simulink model "main"  (R2022b)
settings: Solver=FixedStepDiscrete  StartTime=0.0  StopTime=2000  FixedStep=0.1  RelTol=1e-3
libraries: simulink x3
settings Model: Creator=86134  LastModifiedBy=86134

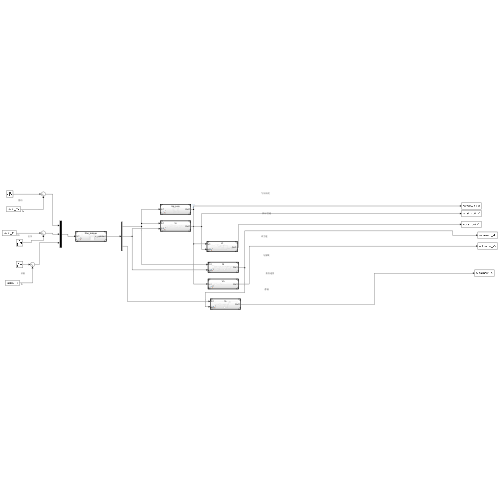
[thumbnail: Simulink's stored preview of the top-level diagram]
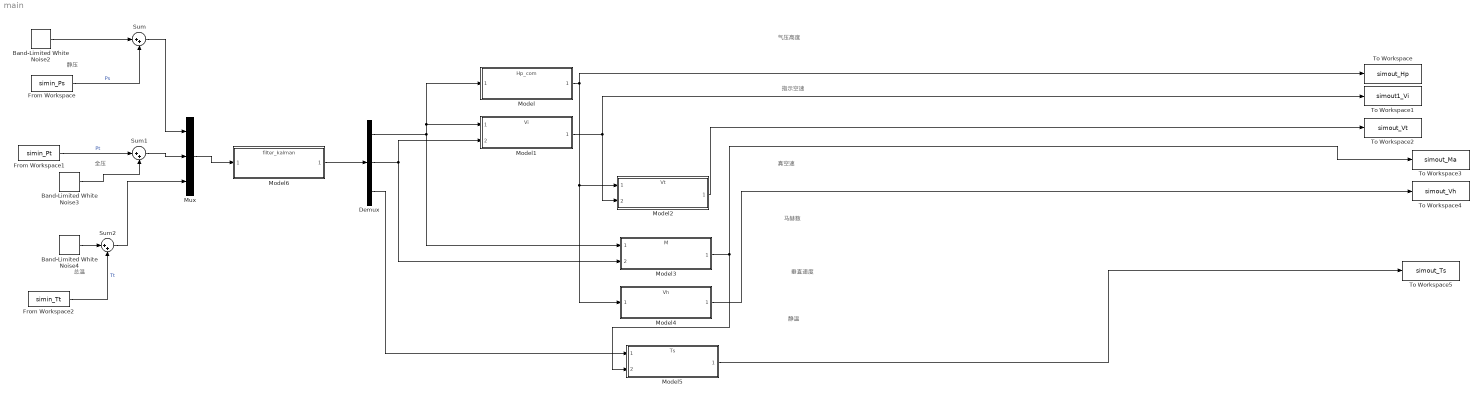
== system main ==
  note: 静温
  note: 垂直速度
  note: 马赫数
  note: 真空速
  note: 指示空速
  note: 气压高度
  note: 总温
  note: 全压
  note: 静压
  Band-Limited White Noise2 : simulink/Sources/Band-Limited White Noise  Cov=0  Ts=0.1  seed=[23341]
  Band-Limited White Noise3 : simulink/Sources/Band-Limited White Noise  Cov=0  Ts=0.1  seed=[23342]
  Band-Limited White Noise4 : simulink/Sources/Band-Limited White Noise  Cov=0  Ts=0.1  seed=[23343]
  Demux : Demux  Outputs=3
  From Workspace : FromWorkspace  VariableName=simin_Ps  SampleTime=0.1
  From Workspace1 : FromWorkspace  VariableName=simin_Pt  SampleTime=0.1
  From Workspace2 : FromWorkspace  VariableName=simin_Tt  SampleTime=0.1
  Model : ModelReference  ModelNameDialog=Hp_com.slx  SimulationMode=Normal  ModelReferenceVersion=1.9
  Model1 : ModelReference  ModelNameDialog=Vi.slx  SimulationMode=Normal  ModelReferenceVersion=1.6
  Model2 : ModelReference  ModelNameDialog=Vt.slx  SimulationMode=Normal  ModelReferenceVersion=1.3
  Model3 : ModelReference  ModelNameDialog=M.slx  SimulationMode=Normal  ModelReferenceVersion=1.5
  Model4 : ModelReference  ModelNameDialog=Vh.slx  SimulationMode=Normal  ModelReferenceVersion=1.14
  Model5 : ModelReference  ModelNameDialog=Ts.slx  SimulationMode=Normal  ModelReferenceVersion=1.4
  Model6 : ModelReference  ModelNameDialog=filter_kalman.slx  SimulationMode=Normal  ModelReferenceVersion=1.44
  Mux : Mux  Inputs=3
  Sum : Sum  Inputs=|++
  Sum1 : Sum  Inputs=|++
  Sum2 : Sum  Inputs=|++
  To Workspace : ToWorkspace  VariableName=simout_Hp  SaveFormat=Timeseries  SampleTime=0.1
  To Workspace1 : ToWorkspace  VariableName=simout1_Vi  SaveFormat=Timeseries  SampleTime=0.1
  To Workspace2 : ToWorkspace  VariableName=simout_Vt  SaveFormat=Timeseries  SampleTime=0.1
  To Workspace3 : ToWorkspace  VariableName=simout_Ma  SaveFormat=Timeseries  SampleTime=0.1
  To Workspace4 : ToWorkspace  VariableName=simout_Vh  SaveFormat=Timeseries  SampleTime=0.1
  To Workspace5 : ToWorkspace  VariableName=simout_Ts  SaveFormat=Timeseries  SampleTime=0.1
  wires:
  Band-Limited White Noise2/1 -> Sum/1
  From Workspace/1 -> Sum/2  "Ps"
  Band-Limited White Noise3/1 -> Sum1/2
  From Workspace1/1 -> Sum1/1  "Pt"
  Band-Limited White Noise4/1 -> Sum2/1
  From Workspace2/1 -> Sum2/2  "Tt"
  Model/1 -> Model4/1, Model2/1, To Workspace/1
  Model5/1 -> To Workspace5/1
  Model2/1 -> To Workspace2/1
  Model4/1 -> To Workspace4/1
  Model1/1 -> Model2/2, To Workspace1/1
  Model3/1 -> To Workspace3/1, Model5/2
  Sum/1 -> Mux/1
  Sum1/1 -> Mux/2
  Sum2/1 -> Mux/3
  Demux/1 -> Model1/1, Model/1, Model3/1
  Demux/2 -> Model1/2, Model3/2
  Demux/3 -> Model5/1
  Model6/1 -> Demux/1
  Mux/1 -> Model6/1
